simulink library "Batteries_BYD"  (R2025b)
settings: Solver=VariableStepAuto  StartTime=0.0  StopTime=10.0  RelTol=1e-3
undefined symbols (not defined in the file or in its folder): battery_builder_rtmsupport, gcbh
libraries: Batteries_BYD_lib x24
(part 2 of 2)

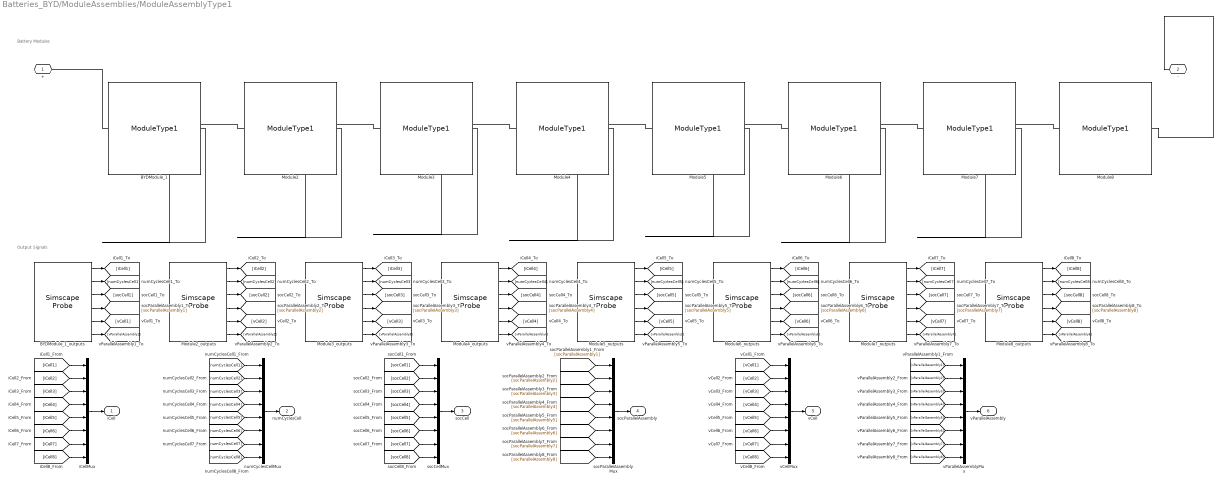
== system Batteries_BYD/ModuleAssemblies/ModuleAssemblyType1 ==
  note: Battery Modules
  note: Output Signals
  BYDModule_1 : Batteries_BYD_lib/Modules/ModuleType1  SOC_vecCell=[0, .01, .02, .03, .04, .05, .06, .07, .08, .09, .1, .11, .12, .13, .14, .15, .16, .17, .18, .19, .2, .21, .22, .23, .24, .25, .26, .27, .28, .29, .3, .31, .32, .33, .34, .35, .36, .37, .38, .39, .4, .41, .42, .43, .44, .45, .46, .47, .48, .49, .5, .51, .52, .53, .54, .55, .56, .57, .58, .59, .6, .61, .62, .63, .64, .65, .66, .67, .68, .69, .7, .71, .72, .73, .74, .75, .76, .77, .78, .79, .8, .81, .82, .83, .84, .85, .86, .87, .88, .89, .9, .91, .92, .93, .94, .95, .96, .97, .98, .99, 1]  V0_vecCell=[2.54959, 2.72277, 2.8309, 2.90338, 2.94932, 2.99568, 3.04282, 3.08893, 3.13237, 3.1748, 3.21261, 3.24735, 3.27811, 3.30611, 3.33207, 3.35348, 3.37373, 3.39078, 3.40552, 3.42083, 3.43203, 3.4417, 3.44978, 3.45814, 3.46654, 3.47495, 3.48258, 3.48961, 3.49665, 3.5042, 3.51255, 3.52116, 3.52942, 3.53684, 3.54421, 3.55146, 3.55892, 3.56648, 3.57366, 3.58054, 3.58765, 3.59465, 3.60064, 3.60661, 3.61259, 3.61852, 3.62445, 3.63043, 3.63671, 3.64314, 3.64971, 3.6568, 3.66398, 3.67131, 3.67896, 3.68659, 3.69422, 3.70211, 3.70999, 3.71791, 3.72583, 3.73426, 3.74295, 3.75164, 3.76009, 3.76809, 3.77609, 3.78411, 3.79209, 3.79975, 3.80711, 3.81469, 3.82306, 3.83141, 3.83964, 3.8465, 3.85319, 3.85997, 3.86692, 3.87404, 3.88116, 3.889, 3.89764, 3.90628, 3.91468, 3.92424, 3.93459, 3.94495, 3.9552, 3.96544, 3.97573, 3.98567, 3.99568, 4.00621, 4.01675, 4.02606, 4.03387, 4.0415, 4.04823, 4.05702, 4.18791] V  V_rangeCell=[2.25, Inf] V  R0_vecCell=[.14748, .16286, .15506, .13564, .11292, .10209, .09565, .09242, .09015, .08876, .08936, .08943, .08993, .0901, .0913, .09117, .0919, .09161, .09109, .09139, .09028, .08916, .08754, .08684, .08616, .08548, .0845, .08334, .08219, .08142, .08122, .08111, .08093, .08056, .08016, .07973, .07949, .07936, .07909, .07879, .07858, .07833, .07771, .07707, .07642, .07575, .07508, .07428, .07341, .07268, .0721, .07169, .07133, .07104, .07087, .07055, .07024, .07001, .06918, .06824, .06729, .06688, .06676, .06663, .06644, .06614, .06584, .06556, .06546, .06525, .065, .06492, .06518, .06543, .06567, .0654, .06507, .06475, .0645, .06431, .06412, .06422, .06463, .06503, .0651, .06525, .06551, .06577, .06603, .06629, .0665, .06632, .06616, .06636, .06665, .06648, .06536, .06416, .06143, .05804, .02838] Ohm  AHCell=3.008 A*hr  extrapolation_optionCell=simscape.enum.extrapolation.nearest  P=6  S=1  iCell_specify=off  iCell_priority=None  iCell=0 A  iCell_nominal_specify=off  iCell_nominal_value=1  iCell_nominal_unit=A  vCell_specify=off  vCell_priority=None  vCell=0 V  vCell_nominal_specify=off  vCell_nominal_value=1  vCell_nominal_unit=V  socCell_specify=off  socCell_priority=High  socCell=1  socCell_nominal_specify=off  socCell_nominal_value=1  socCell_nominal_unit=1  numCyclesCell_specify=off  numCyclesCell_priority=High  numCyclesCell=0  numCyclesCell_nominal_specify=off  numCyclesCell_nominal_value=1  numCyclesCell_nominal_unit=1  vParallelAssembly_specify=off  vParallelAssembly_priority=None  vParallelAssembly=0 V  vParallelAssembly_nominal_specify=off  vParallelAssembly_nominal_value=1  vParallelAssembly_nominal_unit=V  socParallelAssembly_specify=off  socParallelAssembly_priority=None  socParallelAssembly=1  socParallelAssembly_nominal_specify=off  socParallelAssembly_nominal_value=1  socParallelAssembly_nominal_unit=1
      settings: InternalSimscapePortConfiguration="{\"Bottom\":[{\"id\":\"n\",\"label\":\"-\",\"type\":\"foundation.electrical.electrical\"}],\"Left\":[],\"Right\":[],\"Top\":[{\"id\":\"p\",\"label\":\"+\",\"type\":\"foundation.electrical.electrical\"}]}"
  BYDModule_1_outputs : SimscapeProbe  BoundBlock=3  Variables="{\"iCell\":{\"Probing\":\"ON\"},\"numCyclesCell\":{\"Probing\":\"ON\"},\"socCell\":{\"Probing\":\"ON\"},\"socParallelAssembly\":{\"Probing\":\"ON\"},\"vCell\":{\"Probing\":\"ON\"},\"vParallelAssembly\":{\"Probing\":\"ON\"}}"
  Module{2..8} (7 alike) : Batteries_BYD_lib/Modules/ModuleType1  SOC_vecCell=[0, .01, .02, .03, .04, .05, .06, .07, .08, .09, .1, .11, .12, .13, .14, .15, .16, .17, .18, .19, .2, .21, .22, .23, .24, .25, .26, .27, .28, .29, .3, .31, .32, .33, .34, .35, .36, .37, .38, .39, .4, .41, .42, .43, .44, .45, .46, .47, .48, .49, .5, .51, .52, .53, .54, .55, .56, .57, .58, .59, .6, .61, .62, .63, .64, .65, .66, .67, .68, .69, .7, .71, .72, .73, .74, .75, .76, .77, .78, .79, .8, .81, .82, .83, .84, .85, .86, .87, .88, .89, .9, .91, .92, .93, .94, .95, .96, .97, .98, .99, 1]  V0_vecCell=[2.54959, 2.72277, 2.8309, 2.90338, 2.94932, 2.99568, 3.04282, 3.08893, 3.13237, 3.1748, 3.21261, 3.24735, 3.27811, 3.30611, 3.33207, 3.35348, 3.37373, 3.39078, 3.40552, 3.42083, 3.43203, 3.4417, 3.44978, 3.45814, 3.46654, 3.47495, 3.48258, 3.48961, 3.49665, 3.5042, 3.51255, 3.52116, 3.52942, 3.53684, 3.54421, 3.55146, 3.55892, 3.56648, 3.57366, 3.58054, 3.58765, 3.59465, 3.60064, 3.60661, 3.61259, 3.61852, 3.62445, 3.63043, 3.63671, 3.64314, 3.64971, 3.6568, 3.66398, 3.67131, 3.67896, 3.68659, 3.69422, 3.70211, 3.70999, 3.71791, 3.72583, 3.73426, 3.74295, 3.75164, 3.76009, 3.76809, 3.77609, 3.78411, 3.79209, 3.79975, 3.80711, 3.81469, 3.82306, 3.83141, 3.83964, 3.8465, 3.85319, 3.85997, 3.86692, 3.87404, 3.88116, 3.889, 3.89764, 3.90628, 3.91468, 3.92424, 3.93459, 3.94495, 3.9552, 3.96544, 3.97573, 3.98567, 3.99568, 4.00621, 4.01675, 4.02606, 4.03387, 4.0415, 4.04823, 4.05702, 4.18791] V  V_rangeCell=[2.25, Inf] V  R0_vecCell=[.14748, .16286, .15506, .13564, .11292, .10209, .09565, .09242, .09015, .08876, .08936, .08943, .08993, .0901, .0913, .09117, .0919, .09161, .09109, .09139, .09028, .08916, .08754, .08684, .08616, .08548, .0845, .08334, .08219, .08142, .08122, .08111, .08093, .08056, .08016, .07973, .07949, .07936, .07909, .07879, .07858, .07833, .07771, .07707, .07642, .07575, .07508, .07428, .07341, .07268, .0721, .07169, .07133, .07104, .07087, .07055, .07024, .07001, .06918, .06824, .06729, .06688, .06676, .06663, .06644, .06614, .06584, .06556, .06546, .06525, .065, .06492, .06518, .06543, .06567, .0654, .06507, .06475, .0645, .06431, .06412, .06422, .06463, .06503, .0651, .06525, .06551, .06577, .06603, .06629, .0665, .06632, .06616, .06636, .06665, .06648, .06536, .06416, .06143, .05804, .02838] Ohm  AHCell=3.008 A*hr  extrapolation_optionCell=simscape.enum.extrapolation.nearest  P=6  S=1  iCell_specify=off  iCell_priority=None  iCell=0 A  iCell_nominal_specify=off  iCell_nominal_value=1  iCell_nominal_unit=A  vCell_specify=off  vCell_priority=None  vCell=0 V  vCell_nominal_specify=off  vCell_nominal_value=1  vCell_nominal_unit=V  socCell_specify=off  socCell_priority=High  socCell=1  socCell_nominal_specify=off  socCell_nominal_value=1  socCell_nominal_unit=1  numCyclesCell_specify=off  numCyclesCell_priority=High  numCyclesCell=0  numCyclesCell_nominal_specify=off  numCyclesCell_nominal_value=1  numCyclesCell_nominal_unit=1  vParallelAssembly_specify=off  vParallelAssembly_priority=None  vParallelAssembly=0 V  vParallelAssembly_nominal_specify=off  vParallelAssembly_nominal_value=1  vParallelAssembly_nominal_unit=V  socParallelAssembly_specify=off  socParallelAssembly_priority=None  socParallelAssembly=1  socParallelAssembly_nominal_specify=off  socParallelAssembly_nominal_value=1  socParallelAssembly_nominal_unit=1
      settings: InternalSimscapePortConfiguration="{\"Bottom\":[{\"id\":\"n\",\"label\":\"-\",\"type\":\"foundation.electrical.electrical\"}],\"Left\":[],\"Right\":[],\"Top\":[{\"id\":\"p\",\"label\":\"+\",\"type\":\"foundation.electrical.electrical\"}]}"
  Module2_outputs : SimscapeProbe  BoundBlock=4  Variables="{\"iCell\":{\"Probing\":\"ON\"},\"numCyclesCell\":{\"Probing\":\"ON\"},\"socCell\":{\"Probing\":\"ON\"},\"socParallelAssembly\":{\"Probing\":\"ON\"},\"vCell\":{\"Probing\":\"ON\"},\"vParallelAssembly\":{\"Probing\":\"ON\"}}"
  Module3_outputs : SimscapeProbe  BoundBlock=5  Variables="{\"iCell\":{\"Probing\":\"ON\"},\"numCyclesCell\":{\"Probing\":\"ON\"},\"socCell\":{\"Probing\":\"ON\"},\"socParallelAssembly\":{\"Probing\":\"ON\"},\"vCell\":{\"Probing\":\"ON\"},\"vParallelAssembly\":{\"Probing\":\"ON\"}}"
  Module4_outputs : SimscapeProbe  BoundBlock=6  Variables="{\"iCell\":{\"Probing\":\"ON\"},\"numCyclesCell\":{\"Probing\":\"ON\"},\"socCell\":{\"Probing\":\"ON\"},\"socParallelAssembly\":{\"Probing\":\"ON\"},\"vCell\":{\"Probing\":\"ON\"},\"vParallelAssembly\":{\"Probing\":\"ON\"}}"
  Module5_outputs : SimscapeProbe  BoundBlock=7  Variables="{\"iCell\":{\"Probing\":\"ON\"},\"numCyclesCell\":{\"Probing\":\"ON\"},\"socCell\":{\"Probing\":\"ON\"},\"socParallelAssembly\":{\"Probing\":\"ON\"},\"vCell\":{\"Probing\":\"ON\"},\"vParallelAssembly\":{\"Probing\":\"ON\"}}"
  Module6_outputs : SimscapeProbe  BoundBlock=8  Variables="{\"iCell\":{\"Probing\":\"ON\"},\"numCyclesCell\":{\"Probing\":\"ON\"},\"socCell\":{\"Probing\":\"ON\"},\"socParallelAssembly\":{\"Probing\":\"ON\"},\"vCell\":{\"Probing\":\"ON\"},\"vParallelAssembly\":{\"Probing\":\"ON\"}}"
  Module7_outputs : SimscapeProbe  BoundBlock=9  Variables="{\"iCell\":{\"Probing\":\"ON\"},\"numCyclesCell\":{\"Probing\":\"ON\"},\"socCell\":{\"Probing\":\"ON\"},\"socParallelAssembly\":{\"Probing\":\"ON\"},\"vCell\":{\"Probing\":\"ON\"},\"vParallelAssembly\":{\"Probing\":\"ON\"}}"
  Module8_outputs : SimscapeProbe  BoundBlock=10  Variables="{\"iCell\":{\"Probing\":\"ON\"},\"numCyclesCell\":{\"Probing\":\"ON\"},\"socCell\":{\"Probing\":\"ON\"},\"socParallelAssembly\":{\"Probing\":\"ON\"},\"vCell\":{\"Probing\":\"ON\"},\"vParallelAssembly\":{\"Probing\":\"ON\"}}"
  iCellMux : Mux  Inputs=8
  numCyclesCellMux : Mux  Inputs=8
  socCellMux : Mux  Inputs=8
  socParallelAssemblyMux : Mux  Inputs=8
  vCellMux : Mux  Inputs=8
  vParallelAssemblyMux : Mux  Inputs=8
  + : PMIOPort  Side=Left
  - : PMIOPort  Port=2  Side=Right
  iCell : Outport
  numCyclesCell : Outport  Port=2
  socCell : Outport  Port=3
  socParallelAssembly : Outport  Port=4
  vCell : Outport  Port=5
  vParallelAssembly : Outport  Port=6
  wires:
  BYDModule_1_outputs/1 -> [iCell1]
  iCellMux/1 -> iCell/1
  [iCell1] -> iCellMux/1
  BYDModule_1_outputs/2 -> [numCyclesCell1]
  numCyclesCellMux/1 -> numCyclesCell/1
  [numCyclesCell1] -> numCyclesCellMux/1
  BYDModule_1_outputs/3 -> [socCell1]
  socCellMux/1 -> socCell/1
  [socCell1] -> socCellMux/1
  BYDModule_1_outputs/4 -> [socParallelAssembly1]
  socParallelAssemblyMux/1 -> socParallelAssembly/1
  [socParallelAssembly1] -> socParallelAssemblyMux/1
  BYDModule_1_outputs/5 -> [vCell1]
  vCellMux/1 -> vCell/1
  [vCell1] -> vCellMux/1
  BYDModule_1_outputs/6 -> [vParallelAssembly1]
  vParallelAssemblyMux/1 -> vParallelAssembly/1
  [vParallelAssembly1] -> vParallelAssemblyMux/1
  Module2_outputs/1 -> [iCell2]
  [iCell2] -> iCellMux/2
  Module2_outputs/2 -> [numCyclesCell2]
  [numCyclesCell2] -> numCyclesCellMux/2
  Module2_outputs/3 -> [socCell2]
  [socCell2] -> socCellMux/2
  Module2_outputs/4 -> [socParallelAssembly2]
  [socParallelAssembly2] -> socParallelAssemblyMux/2
  Module2_outputs/5 -> [vCell2]
  [vCell2] -> vCellMux/2
  Module2_outputs/6 -> [vParallelAssembly2]
  [vParallelAssembly2] -> vParallelAssemblyMux/2
  Module3_outputs/1 -> [iCell3]
  [iCell3] -> iCellMux/3
  Module3_outputs/2 -> [numCyclesCell3]
  [numCyclesCell3] -> numCyclesCellMux/3
  Module3_outputs/3 -> [socCell3]
  [socCell3] -> socCellMux/3
  Module3_outputs/4 -> [socParallelAssembly3]
  [socParallelAssembly3] -> socParallelAssemblyMux/3
  Module3_outputs/5 -> [vCell3]
  [vCell3] -> vCellMux/3
  Module3_outputs/6 -> [vParallelAssembly3]
  [vParallelAssembly3] -> vParallelAssemblyMux/3
  Module4_outputs/1 -> [iCell4]
  [iCell4] -> iCellMux/4
  Module4_outputs/2 -> [numCyclesCell4]
  [numCyclesCell4] -> numCyclesCellMux/4
  Module4_outputs/3 -> [socCell4]
  [socCell4] -> socCellMux/4
  Module4_outputs/4 -> [socParallelAssembly4]
  [socParallelAssembly4] -> socParallelAssemblyMux/4
  Module4_outputs/5 -> [vCell4]
  [vCell4] -> vCellMux/4
  Module4_outputs/6 -> [vParallelAssembly4]
  [vParallelAssembly4] -> vParallelAssemblyMux/4
  Module5_outputs/1 -> [iCell5]
  [iCell5] -> iCellMux/5
  Module5_outputs/2 -> [numCyclesCell5]
  [numCyclesCell5] -> numCyclesCellMux/5
  Module5_outputs/3 -> [socCell5]
  [socCell5] -> socCellMux/5
  Module5_outputs/4 -> [socParallelAssembly5]
  [socParallelAssembly5] -> socParallelAssemblyMux/5
  Module5_outputs/5 -> [vCell5]
  [vCell5] -> vCellMux/5
  Module5_outputs/6 -> [vParallelAssembly5]
  [vParallelAssembly5] -> vParallelAssemblyMux/5
  Module6_outputs/1 -> [iCell6]
  [iCell6] -> iCellMux/6
  Module6_outputs/2 -> [numCyclesCell6]
  [numCyclesCell6] -> numCyclesCellMux/6
  Module6_outputs/3 -> [socCell6]
  [socCell6] -> socCellMux/6
  Module6_outputs/4 -> [socParallelAssembly6]
  [socParallelAssembly6] -> socParallelAssemblyMux/6
  Module6_outputs/5 -> [vCell6]
  [vCell6] -> vCellMux/6
  Module6_outputs/6 -> [vParallelAssembly6]
  [vParallelAssembly6] -> vParallelAssemblyMux/6
  Module7_outputs/1 -> [iCell7]
  [iCell7] -> iCellMux/7
  Module7_outputs/2 -> [numCyclesCell7]
  [numCyclesCell7] -> numCyclesCellMux/7
  Module7_outputs/3 -> [socCell7]
  [socCell7] -> socCellMux/7
  Module7_outputs/4 -> [socParallelAssembly7]
  [socParallelAssembly7] -> socParallelAssemblyMux/7
  Module7_outputs/5 -> [vCell7]
  [vCell7] -> vCellMux/7
  Module7_outputs/6 -> [vParallelAssembly7]
  [vParallelAssembly7] -> vParallelAssemblyMux/7
  Module8_outputs/1 -> [iCell8]
  [iCell8] -> iCellMux/8
  Module8_outputs/2 -> [numCyclesCell8]
  [numCyclesCell8] -> numCyclesCellMux/8
  Module8_outputs/3 -> [socCell8]
  [socCell8] -> socCellMux/8
  Module8_outputs/4 -> [socParallelAssembly8]
  [socParallelAssembly8] -> socParallelAssemblyMux/8
  Module8_outputs/5 -> [vCell8]
  [vCell8] -> vCellMux/8
  Module8_outputs/6 -> [vParallelAssembly8]
  [vParallelAssembly8] -> vParallelAssemblyMux/8
  connections:
  Module2/LConn1 -- BYDModule_1/RConn1
  Module3/LConn1 -- Module2/RConn1
  Module4/LConn1 -- Module3/RConn1
  Module5/LConn1 -- Module4/RConn1
  Module6/LConn1 -- Module5/RConn1
  Module7/LConn1 -- Module6/RConn1
  Module8/LConn1 -- Module7/RConn1
  BYDModule_1/LConn1 -- +/RConn1
  Module8/RConn1 -- -/RConn1
